simulink model "autosar_subcomponent"  (R2022b)
settings: Solver=FixedStepDiscrete  StartTime=0.0  StopTime=10.0  RelTol=1e-3
model workspace (MATLAB code in the model file + MAT data in the model file):
  cmdLim = Simulink.Parameter
  cmdLim.Value = 15
  cmdLim.Description = 'Limit for controlling the maximum surface command angle.'
  cmdLim.Min = 0
  cmdLim.Max = 90
  cmdLim.DocUnits = 'deg'
  dispGain = Simulink.Parameter
  dispGain.Value = 0.75
  dispGain.Description = 'Gain applied to the displacement error.'
  dispGain.Min = 0
  dispGain.Max = []
  dispGain.DocUnits = 'deg/sec/deg'
  dispLim = Simulink.Parameter
  dispLim.Value = 30
  dispLim.Description = 'Limit for controlling the maximum commanded angle.'
  dispLim.Min = 0
  dispLim.Max = 180
  dispLim.DocUnits = 'deg'
  intGain = Simulink.Parameter
  intGain.Value = 0.5
  intGain.Description = 'Gain applied to the integral error.'
  intGain.Min = 0
  intGain.Max = []
  intGain.DocUnits = 'deg/sec/deg/sec'
  intLim = Simulink.Parameter
  intLim.Value = 5
  intLim.Description = 'Limit for controlling the maximum commanded angle.'
  intLim.Min = 0
  intLim.Max = 90
  intLim.DocUnits = 'deg'
  rateGain = Simulink.Parameter
  rateGain.Value = 2
  rateGain.Description = 'Gain applied to the rate error.'
  rateGain.Min = 0
  rateGain.Max = []
  rateGain.DocUnits = 'deg/deg/sec'
  rateLim = Simulink.Parameter
  rateLim.Value = 6
  rateLim.Description = 'Limit for controlling the maximum commanded angle.'
  rateLim.Min = 0
  rateLim.Max = 180
  rateLim.DocUnits = 'deg/sec'
  hdgGain = Simulink.Parameter
  hdgGain.Value = 0.015
  PressureEstimation = Simulink.LookupTable
  PressureEstimation.Table = Simulink.lookuptable.Table
  PressureEstimation.Table.Value = [0.806253176324 0.553142316929 0.37151500209 0.277667903103 0.220198954207 0.181288665766 0.153200000489 0.115431020872 0.0913067476324 0.0746519188607 0.0625231108324 0.0533383634277 ... (306 elements, 18x17)]
  PressureEstimation.Table.Dimensions = [18 17]
  PressureEstimation.Table.DataType = 'auto'
  PressureEstimation.Table.Min = -1
  PressureEstimation.Table.Max = 100
  PressureEstimation.Table.FieldName = 'Table'
  PressureEstimation.Table.Description = 'Pressure estimation Table data description'
  PressureEstimation.Breakpoints(1) = Simulink.lookuptable.Breakpoint
  PressureEstimation.Breakpoints(1).Value = [50 75 100 125 150 175 200 250 300 350 400 450 500 600 700 800 900 1000]
  PressureEstimation.Breakpoints(1).TunableSizeName = 'N1'
  PressureEstimation.Breakpoints(1).Dimensions = [1 18]
  PressureEstimation.Breakpoints(1).DataType = 'double'
  PressureEstimation.Breakpoints(1).FieldName = 'BP1'
  PressureEstimation.Breakpoints(2) = Simulink.lookuptable.Breakpoint
  PressureEstimation.Breakpoints(2).Value = [0 3 6 9 12 15 18 21 24 27 30 35 46 57 68 79 90]
  PressureEstimation.Breakpoints(2).TunableSizeName = 'N2'
  PressureEstimation.Breakpoints(2).Dimensions = [1 17]
  PressureEstimation.Breakpoints(2).DataType = 'double'
  PressureEstimation.Breakpoints(2).FieldName = 'BP2'
  PressureEstimation.SupportTunableSize = 0
  PressureEstimation.StructTypeInfo = Simulink.lookuptable.StructTypeInfo
  PressureEstimation.StructTypeInfo.Name = 'PressureEstimationType'
  PressureEstimation.StructTypeInfo.DataScope = 'Auto'
  engine_speed = Simulink.Parameter
  engine_speed.Value = 300
  engine_speed.Description = 'Engine Speed'
  engine_speed.DataType = 'double'
  engine_speed.Min = 100
  engine_speed.Max = 1000
  engine_speed.Complexity = 'real'
  engine_speed.Dimensions = [1 1]
  max_press = Simulink.Parameter
  max_press.Value = 0.95
  max_press.Description = 'Maximum Pressure'
  max_press.DataType = 'double'
  max_press.Min = 0
  max_press.Max = 1
  max_press.DocUnits = 'm'
  max_press.Complexity = 'real'
  max_press.Dimensions = [1 1]
  max_speed = Simulink.Parameter
  max_speed.Value = 300
  max_speed.Description = 'Maximum Speed'
  max_speed.DataType = 'double'
  max_speed.Min = 0
  max_speed.Max = 1000
  max_speed.DocUnits = 'm/N'
  max_speed.Complexity = 'real'
  max_speed.Dimensions = [1 1]
settings Model: RequirementInfo={} %GIDa_fe9045fd_0412_4b6e_8206_617cc20e6fde  FPTRunName=Active  ParameterArgumentNames=PressureEstimation,engine_speed,max_press,max_speed  Creator=The MathWorks, Inc.  LastModifiedBy=The MathWorks, Inc.
settings SolverCC: AlgebraicLoopSolver=TrustRegion  AutoInsertRateTranBlk=on  MaxZcPerStep=1
settings DataIOCC: SaveOutput=off  SignalLogging=off  DSMLogging=off  SaveTime=off  ReturnWorkspaceOutputs=off
settings OptimizationCC: DefaultParameterBehavior=Inlined  UseDivisionForNetSlopeComputation=on  UseFloatMulNetSlope=on  UseSpecifiedMinMax=on  InlineInvariantSignals=on  EnhancedBackFolding=on  PassReuseOutputArgsAs=Individual arguments  ZeroExternalMemoryAtStartup=off  ZeroInternalMemoryAtStartup=off  NoFixptDivByZeroProtection=on  EfficientFloat2IntCast=on  OptimizeBlockOrder=speed  DifferentSizesBufferReuse=on  OptimizationCustomize=off  EfficientTunableParamExpr=on
settings DebuggingCC: ParameterTunabilityLossMsg=error  UnconnectedInputMsg=warning  UnconnectedOutputMsg=warning  UnconnectedLineMsg=warning  AllowSymbolicDim=off  ModelReferenceSymbolNameMessage=none  SFUnexpectedBacktrackingDiag=warning  SFNoUnconditionalDefaultTransitionDiag=warning  SFExecutionAtInitializationDiag=none  SFMachineParentedDataDiag=warning  ArithmeticOperatorsInVariantConditions=warning
settings HardwareCC: ProdLongLongMode=on
settings ModelReferenceCC: EnableRefExpFcnMdlSchedulingChecks=on
settings SFSimCC: MATLABDynamicMemAlloc=off
settings RTWCC: Description=AUTOSAR  SystemTargetFile=autosar.tlc  GenCodeOnly=on  TemplateMakefile=ert_default_tmf  GenerateReport=on  RTWVerbose=off  BuildConfiguration=Faster Runs  IncludeHyperlinkInReport=on  LaunchReport=on  GenerateTraceInfo=on  GenerateTraceReport=on  GenerateTraceReportSl=on  GenerateTraceReportSf=on  GenerateTraceReportEml=on  GenerateCodeMetricsReport=on  DLArmComputeVersion=19.05
settings CodeAppCC: ForceParamTrailComments=on  IgnoreCustomStorageClasses=off  OperatorAnnotations=on  SimulinkDataObjDesc=on  SFDataObjDesc=on  CustomSymbolStrGlobalVar=rt$N$M  CustomSymbolStrType=$N$M  CustomSymbolStrFcn=$N$M$F  CustomSymbolStrMacro=$N$M  InsertBlockDesc=on  EnableCustomComments=on  ReqsInCode=on
settings STFCustomTargetCC: TargetLangStandard=C99 (ISO)  MultiwordLength=256  ParMdlRefBuildCompliant=on  CompOptLevelCompliant=on  IncludeMdlTerminateFcn=off  CombineOutputUpdateFcns=on  SuppressErrorStatus=on  ERTCustomFileBanners=on  SupportNonFinite=off  SupportComplex=off  SupportContinuousTime=off  SupportNonInlinedSFcns=off  RemoveResetFunc=on  MATLABClassNameForMDSCustomization=Simulink.SoftwareTarget.ERTCustomization  CPPClassGenCompliant=on  AutosarCompliant=on  UseToolchainInfoCompliant=on  LookupTableObjectStructAxisOrder=2,1,3,4,...  LUTObjectStructOrderEvenSpacing=Size,Table,Breakpoints  SystemTargetFile=autosar.tlc
settings ERTTargetCC: TargetLangStandard=C99 (ISO)  ConcurrentExecutionCompliant=off  IncludeMdlTerminateFcn=off  SuppressErrorStatus=on  SupportNonFinite=off  SupportComplex=off  ModelStepFunctionPrototypeControlCompliant=off  AutosarCompliant=on  LookupTableObjectStructAxisOrder=2,1,3,4,...  LUTObjectStructOrderEvenSpacing=Size,Table,Breakpoints  InlinedParameterPlacement=NonHierarchical  ERTCustomFileTemplate=example_file_process.tlc
settings ConfigComp: CovScope=ReferencedModels  CovSaveName=covdata_rollAP  CovMetricSettings=dcmtrwe  CovHTMLOptions=-sRT=1 -aTS=1 -bRG=1 -bTC=1 -hTR=1 -nFC=0 -scm=1 -bcm=1 -xEv=0  CovSaveCumulativeToWorkspaceVar=on  CovSaveSingleToWorkspaceVar=on  CovCumulativeVarName=covCumulativeData_rollAP  CovReportOnPause=off  CovExternalEMLEnable=off  CovSFcnEnable=off

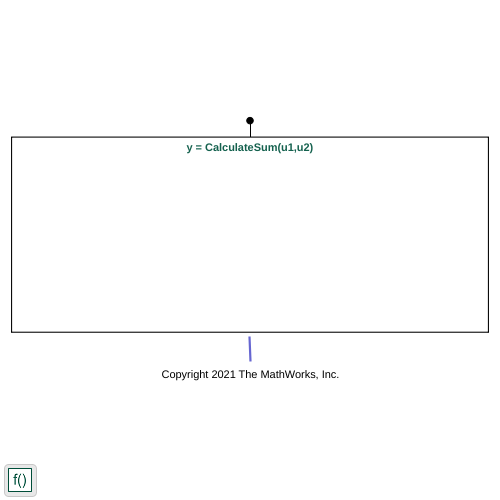
[thumbnail: Simulink's stored preview of the top-level diagram]
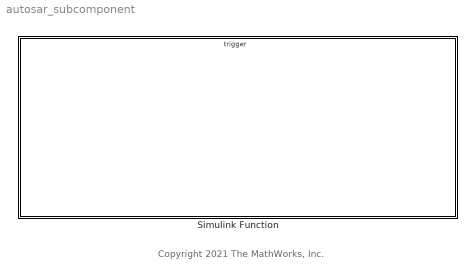
== system autosar_subcomponent ==
  note: Copyright 2021 The MathWorks, Inc.
  Simulink Function : Subsystem  TreatAsAtomicUnit=on

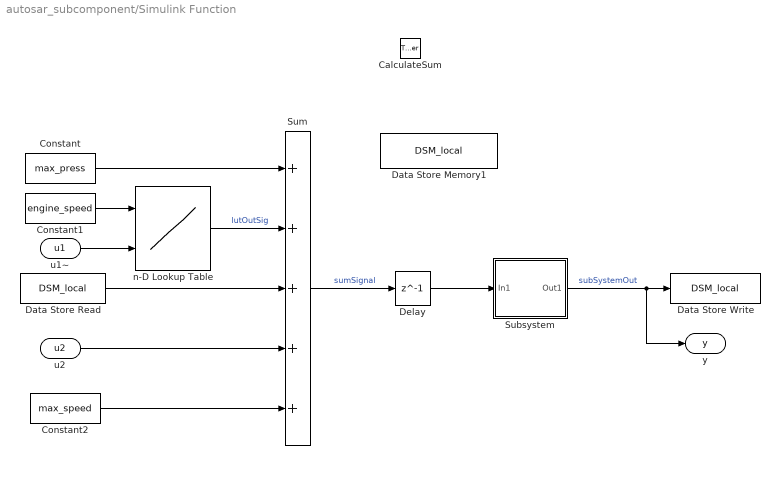
== system autosar_subcomponent/Simulink Function ==
  CalculateSum : TriggerPort  TriggerType=function-call  IsSimulinkFunction=on  FunctionName=CalculateSum  FunctionVisibility=scoped  VariantControl=(inherit)
  Constant : Constant  Value=max_press
  Constant1 : Constant  Value=engine_speed
  Constant2 : Constant  Value=max_speed
  Data Store Memory1 : DataStoreMemory  DataStoreName=DSM_local  ShowAdditionalParam=off  OutDataTypeStr=double
  Data Store Read : DataStoreRead  DataStoreName=DSM_local  IndexOptions=Index vector (dialog)  Indices=1  OutputSizes=1
  Data Store Write : DataStoreWrite  DataStoreName=DSM_local  IndexOptions=Index vector (dialog)  Indices=1  OutputSizes=1
  Delay : Delay  DelayLength=1  InitialCondition=0  StateName=X
  Subsystem : Subsystem  mask{Gain=21}
  Sum : Sum  Inputs=+++++  InputSameDT=on  OutDataTypeStr=Inherit: Same as first input
  n-D Lookup Table : Lookup_n-D  DataSpecification=Lookup table object  LookupTableObject=PressureEstimation  BreakpointsForDimension3=[5, 7]  Table=reshape(repmat([4 5 6;16 19 20;10 18 23],1,2),[3,3,2])  InternalRulePriority=Speed  RndMeth=Simplest
      settings: InputPortMap=u0,u1
  u1~ : ArgIn  DisableCoverage=on  ArgumentName=u1
  u2 : ArgIn  DisableCoverage=on  Port=2  ArgumentName=u2
  y : ArgOut  DisableCoverage=on  ArgumentName=y
  wires:
  Constant2/1 -> Sum/5
  u1~/1 -> n-D Lookup Table/2
  Subsystem/1(Out1) -> y/1, Data Store Write/1  "subSystemOut"
  n-D Lookup Table/1 -> Sum/2  "lutOutSig"
  Data Store Read/1 -> Sum/3
  u2/1 -> Sum/4
  Delay/1 -> Subsystem/1(In1)
  Constant1/1 -> n-D Lookup Table/1
  Constant/1 -> Sum/1
  Sum/1 -> Delay/1  "sumSignal"

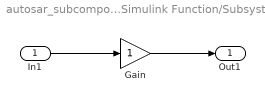
== system autosar_subcomponent/Simulink Function/Subsystem ==
  In1 : Inport
  Gain : Gain
  Out1 : Outport  VectorParamsAs1DForOutWhenUnconnected=off
  wires:
  Gain/1 -> Out1/1
  In1/1 -> Gain/1
